simulink model "InjCtl_qCoSync"  (R2016b)
settings: configuration reference "CodeGenConfigSet" (kept outside this file)
undefined symbols (not defined in the file or in its folder): EngState_conv
libraries: simulink x1
settings Model: Creator=zhoutinglin  LastModifiedBy=zhoutinglin
settings ConfigSetRef: SourceLocation=Base Workspace

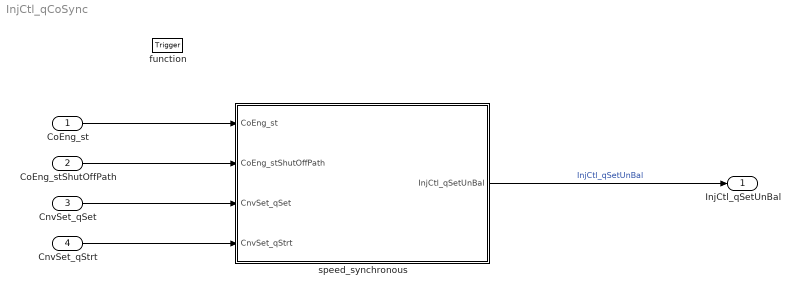
== system InjCtl_qCoSync ==
  CoEng_st : Inport  Description=Engine coordinator state  OutDataTypeStr=Enum: EngState_conv
  CoEng_stShutOffPath : Inport  Description=Active shut-off paths resulting from active reversible,irreversible and afterrun shut-off paths  Port=2  OutMin=0  OutMax=65535  OutDataTypeStr=State_uint16
  CnvSet_qSet : Inport  Tag=mg/hub  Description=Set point injection quantity  Port=3  OutMin=-319  OutMax=319  OutDataTypeStr=FuelMass_mg_hub
  CnvSet_qStrt : Inport  Tag=mg/hub  Description=Injection start quantity  Port=4  OutMin=-319  OutMax=319  OutDataTypeStr=FuelMass_mg_hub
  function : TriggerPort  TriggerType=function-call  VariantControl=Variant
  " speed_synchronous" : Subsystem
  InjCtl_qSetUnBal : Outport  Tag=mg/hub  Description=Current injection quantity  OutMin=-319  OutMax=319  OutDataTypeStr=FuelMass_mg_hub
  wires:
  " speed_synchronous"/1(InjCtl_qSetUnBal) -> InjCtl_qSetUnBal/1  "InjCtl_qSetUnBal"
  CoEng_st/1 -> " speed_synchronous"/1(CoEng_st)
  CnvSet_qStrt/1 -> " speed_synchronous"/4(CnvSet_qStrt)
  CnvSet_qSet/1 -> " speed_synchronous"/3(CnvSet_qSet)
  CoEng_stShutOffPath/1 -> " speed_synchronous"/2(CoEng_stShutOffPath)

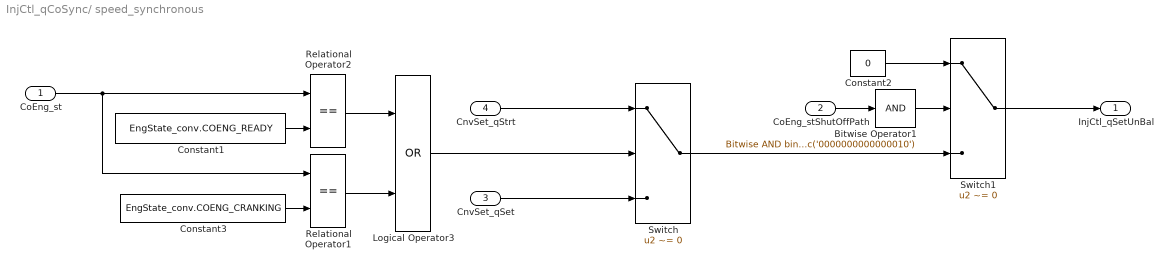
== system InjCtl_qCoSync/ speed_synchronous ==
  CoEng_st : Inport
  CoEng_stShutOffPath : Inport  Port=2
  CnvSet_qSet : Inport  Port=3
  CnvSet_qStrt : Inport  Port=4
  Bitwise Operator1 : simulink/Logic and Bit Operations/Bitwise Operator  logicop=AND  UseBitMask=on  BitMask=bin2dec('0000000000000010')  BitMaskRealWorld=Stored Integer
  Constant1 : Constant  Value=EngState_conv.COENG_READY
  Constant2 : Constant  Value=0  OutDataTypeStr=Inherit: Inherit via back propagation
  Constant3 : Constant  Value=EngState_conv.COENG_CRANKING
  Logical Operator3 : Logic  Operator=OR  AllPortsSameDT=off  OutDataTypeStr=boolean
  Relational Operator1 : RelationalOperator  Operator===  OutDataTypeStr=boolean  RndMeth=Simplest  InputSameDT=on
  Relational Operator2 : RelationalOperator  Operator===  OutDataTypeStr=boolean  RndMeth=Simplest  InputSameDT=on
  Switch : Switch  Criteria=u2 ~= 0  OutDataTypeStr=Inherit: Inherit via back propagation  SaturateOnIntegerOverflow=on  InputSameDT=on
  Switch1 : Switch  Criteria=u2 ~= 0  OutDataTypeStr=Inherit: Inherit via back propagation  SaturateOnIntegerOverflow=on  InputSameDT=on
  InjCtl_qSetUnBal : Outport
  wires:
  Logical Operator3/1 -> Switch/2
  Bitwise Operator1/1 -> Switch1/2
  Switch1/1 -> InjCtl_qSetUnBal/1
  CoEng_stShutOffPath/1 -> Bitwise Operator1/1
  Constant2/1 -> Switch1/1
  CnvSet_qSet/1 -> Switch/3
  CnvSet_qStrt/1 -> Switch/1
  Relational Operator2/1 -> Logical Operator3/1
  Constant1/1 -> Relational Operator2/2
  Relational Operator1/1 -> Logical Operator3/2
  CoEng_st/1 -> Relational Operator2/1, Relational Operator1/1
  Constant3/1 -> Relational Operator1/2
  Switch/1 -> Switch1/3
